simulink model "pure_pursuit"  (R2025b)
settings: Solver=VariableStepAuto  StartTime=0.0  StopTime=40  RelTol=1e-3
libraries: robotmobilelib x2, autolibshared x1
settings Model: Creator=omer  LastModifiedBy=omer

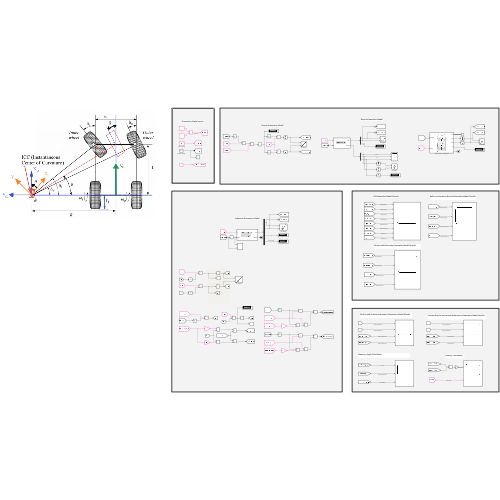
[thumbnail: Simulink's stored preview of the top-level diagram]
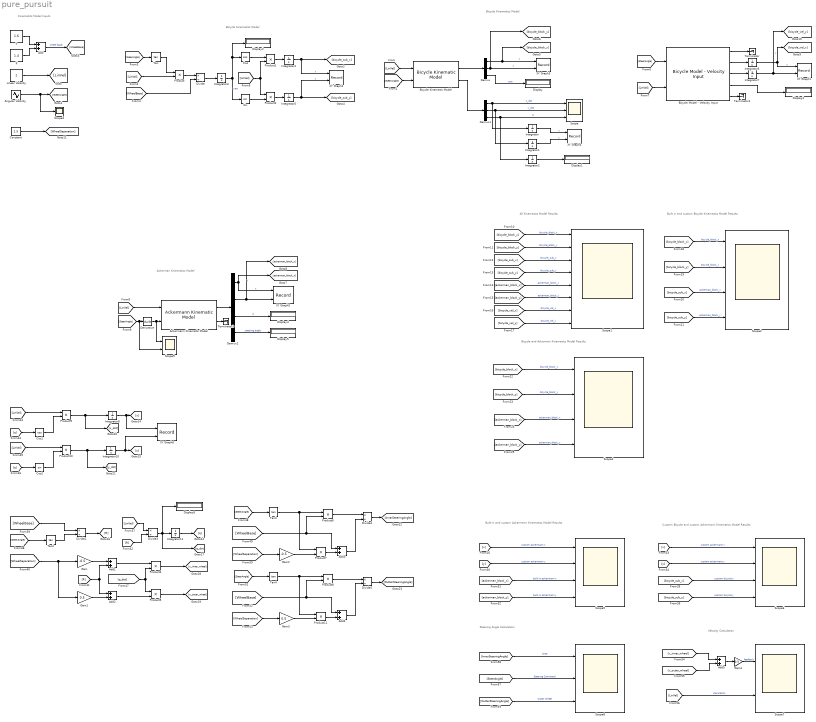
== system pure_pursuit ==
  note: Bicycle Kinematics Model
  note: Bicycle Kinematics Model
  note: Ackerman Kinematics Model
  note: Kinematics Model Inputs
  note: All Kinematics Model Results
  note: Built in and custom Bicycle Kinematics Model Results
  note: Bicycle and Ackerman Kinematics Model Results
  note: Built-in and custom Ackermann Kinematics Model Results
  note: Custom Bicycle and custom Ackermann Kinematics Model Results
  note: Velocity Calculation
  note: Steering Angle Calculation
  Ackermann Kinematic Model : robotmobilelib/Ackermann Kinematic Model  WheelBase=3  VehicleSpeedRange=[-10 10]  MaxSteeringAngle=pi/4  InitialState=[0; 0; 0; 0]  SimulateUsing=Interpreted execution
  Add{,1..5} (6 alike) : Sum
  Angular Velocity : Sin  Amplitude=0.6  Frequency=0.2  SampleTime=0
  Bicycle Kinematic Model : robotmobilelib/Bicycle Kinematic Model  VehicleInputs=Vehicle Speed & Steering Angle  WheelBase=3  VehicleSpeedRange=[-10 10]  MaxSteeringAngle=pi/4  InitialState=[0; 0; 0]  SimulateUsing=Interpreted execution
  Bicycle Model - Velocity Input : autolibshared/Bicycle Model - Velocity Input  trackMode=Single (bicycle)  inputMode=External longitudinal velocity  frontSteerMode=on  rearSteerMode=off  windMode=off  muMode=off  extFMode=off  extMMode=off  aMode=2  NF=2  NR=2  m=2000  a=1.4  b=1.6  h=0.35  X_o=0  xdot_o=0  CalphaMode=off  sigmaMode=on  w=[1.4,1.4]  Cy_f=12e3  Cy_r=11e3  sigma_f=.1  sigma_r=.1  alpha_f_brk=[-.1 .1]  Cy_f_data=[-9e3 9e3]  alpha_r_brk=[-.1 .1]  Cy_r_data=[-9e3 9e3]  Y_o=0  ydot_o=0  Izz=4000  psi_o=0  r_o=0  Af=2  Cd=.3  Cl=.1  Cpm=.1  beta_w=[0 0.01:0.01:0.3]  Cs=[0 0.01:0.01:0.3]  Cym=[0 1e-6:0.01:0.3]  Pabs=101325  Tair=273  g=9.81  mu=1  xdot_tol=.01  Fznom=5000  Fxtire_sat=1e6  Fytire_sat=1e6  longOff=0  latOff=0  vertOff=0
      settings: LibrarySourceBlock=vehdynlibeom/Bicycle Model - Velocity Input
  Constant : Constant  Value=2.5
  Cos : Trigonometry  Operator=cos
  Cos1 : Trigonometry  Operator=cos
  Cos2 : Trigonometry
  Demux : Demux  Outputs=3
  Demux1 : Demux  Outputs=3
  Demux2 : Demux
  Derivative : Derivative
  Display{,1..5,8} (7 alike) : Display
  Divide{,2..5} (5 alike) : Product  Inputs=*/
  Gain : Gain  Gain=-0.5
  Gain1 : Gain  Gain=0.5
  Gain2 : Gain  Gain=-0.5
  Gain3 : Gain  Gain=0.5
  Gain4 : Gain  Gain=0.5
  Integrator{,1..8,10..11} (11 alike) : Integrator
  Linear Velocity : Constant
  Product{,1..2,4..11} (11 alike) : Product
  Scope : Scope  NumInputPorts=3
      settings: ActiveDisplayYMinimum=-1  ActiveDisplayYMaximum=1
  Scope1 : Scope  NumInputPorts=8
      settings: ActiveDisplayYMinimum=-7.1617442519403234  ActiveDisplayYMaximum=20.38246591713515
  Scope{2,4..6} (4 alike) : Scope  NumInputPorts=4
      Scope2 settings: ActiveDisplayYMinimum=0.32572897203293749  ActiveDisplayYMaximum=21.907338374210166  DataLoggingVariableName=ScopeData2
      Scope4 settings: ActiveDisplayYMinimum=32.57770845291958  ActiveDisplayYMaximum=624.63304863060557  DataLoggingVariableName=ScopeData4
      Scope5 settings: ActiveDisplayYMinimum=-4.3902728806219606  ActiveDisplayYMaximum=29.013832851375891  DataLoggingVariableName=ScopeData5
      Scope6 settings: ActiveDisplayYMinimum=-3.4268970997372428  ActiveDisplayYMaximum=28.386536930736913  DataLoggingVariableName=ScopeData6
  Scope3 : Scope
      settings: ActiveDisplayYMinimum=-1.3341695524882851  ActiveDisplayYMaximum=1.7529271348584103  DataLoggingVariableName=ScopeData3
  Scope7 : Scope  NumInputPorts=2
      settings: ActiveDisplayYMinimum=-3.4268970997372428  ActiveDisplayYMaximum=28.386536930736913  DataLoggingVariableName=ScopeData7
  Scope8 : Scope  NumInputPorts=3
      settings: ActiveDisplayYMinimum=-4.3617646340530536  ActiveDisplayYMaximum=11.80186087051403  DataLoggingVariableName=ScopeData8
  Scope9 : Scope  NumInputPorts=2
      settings: ActiveDisplayYMinimum=-1.3341695524882851  ActiveDisplayYMaximum=1.7529271348584103  DataLoggingVariableName=ScopeData9
  Sin : Trigonometry
  Tan{,2..4} (4 alike) : Trigonometry  Operator=tan
  Terminator : Terminator
  Terminator1 : Terminator
  Terminator3 : Terminator
  XY Graph1 : Record  NumPorts=2.0  FileSettingsInternal="{\"entries\":[{\"content\":{\"excelSettings\":{\"content\":{},\"type\":\"Streamout.ExcelSettings\"},\"parquetSettings\":{\"content\":{},\"type\":\"Streamout.ParquetSettings\"}},\"type\":\"Streamout.FileSettingStorage\",\"uuid\":\"\"}],\"packageUris\":[\"http:\\/\\/schema.mathworks.com\\/mf0\\/streamout_blocks\\/R2020a\"],\"version\":\"1.0\"}"  FrameSettings=[0, 0]  Layout=[1 1]  SignalsInternal="{\"entries\":[{\"content\":{\"signals\":[{\"content\":{\"blockPath\":[],\"dimensions\":[1],\"domain\":\"\",\"lineColor\":\"#a2142f\",\"lineWidth\":2,\"plots\":[ 1 ],\"port\":1,\"sid\":[\"\"],\"signalID\":1,\"signalName\":\"x\"},\"type\":\"RecordBlkView.Signal\",\"uuid\":\"\"},{\"content\":{\"blockPath\":[],\"dimensions\":[1],\"domain\":\"\",\"lineColor\":\"#139fff\",\"lineWidth\":2,\"plots\":[ 1 ],\"port\":2,\"sid\":[\"\"],\"signalID\":2,\"signalName\":\"y\"},\"type\":\"RecordBlkView.Signal\",\"uuid\":\"\"}]},\"type\":\"RecordBlkView.InputSignals\",\"uuid\":\"\"}],\"packageUris\":[\"http:\\/\\/schema.mathworks.com\\/mf0\\/streamout_blocks\\/R2020a\"],\"version\":\"1.0\"}"  VisualizationBindings="{\"xyplotplugin\":{\"info\":[{\"series\":[{\"bindingParametersList\":[{\"parameter\":\"X-Axis\",\"signalID\":1,\"signalName\":\"x\"},{\"parameter\":\"Y-Axis\",\"signalID\":2,\"signalName\":\"y\"}],\"seriesID\":0}],\"subplotID\":1}]}}"  CompatibilityTag=XY
  XY Graph2 : Record  NumPorts=2.0  FileSettingsInternal="{\"entries\":[{\"content\":{\"excelSettings\":{\"content\":{},\"type\":\"Streamout.ExcelSettings\"},\"parquetSettings\":{\"content\":{},\"type\":\"Streamout.ParquetSettings\"}},\"type\":\"Streamout.FileSettingStorage\",\"uuid\":\"\"}],\"packageUris\":[\"http:\\/\\/schema.mathworks.com\\/mf0\\/streamout_blocks\\/R2020a\"],\"version\":\"1.0\"}"  FrameSettings=[0, 0]  Layout=[1 1]  SignalsInternal="{\"entries\":[{\"content\":{\"signals\":[{\"content\":{\"blockPath\":[],\"dimensions\":[1],\"domain\":\"\",\"lineColor\":\"#a2142f\",\"plots\":[ 1 ],\"port\":1,\"sid\":[\"\"],\"signalID\":1,\"signalName\":\"x\"},\"type\":\"RecordBlkView.Signal\",\"uuid\":\"\"},{\"content\":{\"blockPath\":[],\"dimensions\":[1],\"domain\":\"\",\"lineColor\":\"#139fff\",\"plots\":[ 1 ],\"port\":2,\"sid\":[\"\"],\"signalID\":2,\"signalName\":\"y\"},\"type\":\"RecordBlkView.Signal\",\"uuid\":\"\"}]},\"type\":\"RecordBlkView.InputSignals\",\"uuid\":\"\"}],\"packageUris\":[\"http:\\/\\/schema.mathworks.com\\/mf0\\/streamout_blocks\\/R2020a\"],\"version\":\"1.0\"}"  VisualizationBindings="{\"xyplotplugin\":{\"info\":[{\"series\":[{\"bindingParametersList\":[{\"parameter\":\"X-Axis\",\"signalID\":1,\"signalName\":\"x\"},{\"parameter\":\"Y-Axis\",\"signalID\":2,\"signalName\":\"y\"}],\"seriesID\":0}],\"subplotID\":1}]}}"  CompatibilityTag=XY
  XY Graph3 : Record  NumPorts=2.0  FileSettingsInternal="{\"entries\":[{\"content\":{\"excelSettings\":{\"content\":{},\"type\":\"Streamout.ExcelSettings\"},\"parquetSettings\":{\"content\":{},\"type\":\"Streamout.ParquetSettings\"}},\"type\":\"Streamout.FileSettingStorage\",\"uuid\":\"\"}],\"packageUris\":[\"http:\\/\\/schema.mathworks.com\\/mf0\\/streamout_blocks\\/R2020a\"],\"version\":\"1.0\"}"  FrameSettings=[0, 0]  Layout=[1 1]  SignalsInternal="{\"entries\":[{\"content\":{\"signals\":[{\"content\":{\"blockPath\":[],\"dimensions\":[1],\"domain\":\"\",\"lineColor\":\"#a2142f\",\"plots\":[ 1 ],\"port\":1,\"sid\":[\"\"],\"signalID\":1,\"signalName\":\"x\"},\"type\":\"RecordBlkView.Signal\",\"uuid\":\"\"},{\"content\":{\"blockPath\":[],\"dimensions\":[1],\"domain\":\"\",\"lineColor\":\"#139fff\",\"plots\":[ 1 ],\"port\":2,\"sid\":[\"\"],\"signalID\":2,\"signalName\":\"y\"},\"type\":\"RecordBlkView.Signal\",\"uuid\":\"\"}]},\"type\":\"RecordBlkView.InputSignals\",\"uuid\":\"\"}],\"packageUris\":[\"http:\\/\\/schema.mathworks.com\\/mf0\\/streamout_blocks\\/R2020a\"],\"version\":\"1.0\"}"  VisualizationBindings="{\"xyplotplugin\":{\"info\":[{\"series\":[{\"bindingParametersList\":[{\"parameter\":\"X-Axis\",\"signalID\":1,\"signalName\":\"x\"},{\"parameter\":\"Y-Axis\",\"signalID\":2,\"signalName\":\"y\"}],\"seriesID\":0}],\"subplotID\":1}]}}"  CompatibilityTag=XY
  XY Graph4 : Record  NumPorts=2.0  FileSettingsInternal="{\"entries\":[{\"content\":{\"excelSettings\":{\"content\":{},\"type\":\"Streamout.ExcelSettings\"},\"parquetSettings\":{\"content\":{},\"type\":\"Streamout.ParquetSettings\"}},\"type\":\"Streamout.FileSettingStorage\",\"uuid\":\"\"}],\"packageUris\":[\"http:\\/\\/schema.mathworks.com\\/mf0\\/streamout_blocks\\/R2020a\"],\"version\":\"1.0\"}"  FrameSettings=[0, 0]  Layout=[1 1]  SignalsInternal="{\"entries\":[{\"content\":{\"signals\":[{\"content\":{\"blockPath\":[],\"dimensions\":[1],\"domain\":\"\",\"lineColor\":\"#a2142f\",\"lineWidth\":2,\"plots\":[ 1 ],\"port\":1,\"sid\":[\"\"],\"signalID\":1,\"signalName\":\"x\"},\"type\":\"RecordBlkView.Signal\",\"uuid\":\"\"},{\"content\":{\"blockPath\":[],\"dimensions\":[1],\"domain\":\"\",\"lineColor\":\"#139fff\",\"lineWidth\":2,\"plots\":[ 1 ],\"port\":2,\"sid\":[\"\"],\"signalID\":2,\"signalName\":\"y\"},\"type\":\"RecordBlkView.Signal\",\"uuid\":\"\"}]},\"type\":\"RecordBlkView.InputSignals\",\"uuid\":\"\"}],\"packageUris\":[\"http:\\/\\/schema.mathworks.com\\/mf0\\/streamout_blocks\\/R2020a\"],\"version\":\"1.0\"}"  VisualizationBindings="{\"xyplotplugin\":{\"info\":[{\"series\":[{\"bindingParametersList\":[{\"parameter\":\"X-Axis\",\"signalID\":1,\"signalName\":\"x\"},{\"parameter\":\"Y-Axis\",\"signalID\":2,\"signalName\":\"y\"}],\"seriesID\":0}],\"subplotID\":1}]}}"  CompatibilityTag=XY
  XY Graph5 : Record  NumPorts=2.0  FileSettingsInternal="{\"entries\":[{\"content\":{\"excelSettings\":{\"content\":{},\"type\":\"Streamout.ExcelSettings\"},\"parquetSettings\":{\"content\":{},\"type\":\"Streamout.ParquetSettings\"}},\"type\":\"Streamout.FileSettingStorage\",\"uuid\":\"\"}],\"packageUris\":[\"http:\\/\\/schema.mathworks.com\\/mf0\\/streamout_blocks\\/R2020a\"],\"version\":\"1.0\"}"  FrameSettings=[0, 0]  Layout=[1 1]  SignalsInternal="{\"entries\":[{\"content\":{\"signals\":[{\"content\":{\"blockPath\":[],\"dimensions\":[1],\"domain\":\"\",\"lineColor\":\"#a2142f\",\"lineWidth\":2,\"plots\":[ 1 ],\"port\":1,\"sid\":[\"\"],\"signalID\":1,\"signalName\":\"x\"},\"type\":\"RecordBlkView.Signal\",\"uuid\":\"\"},{\"content\":{\"blockPath\":[],\"dimensions\":[1],\"domain\":\"\",\"lineColor\":\"#139fff\",\"plots\":[ 1 ],\"port\":2,\"sid\":[\"\"],\"signalID\":2,\"signalName\":\"y\"},\"type\":\"RecordBlkView.Signal\",\"uuid\":\"\"}]},\"type\":\"RecordBlkView.InputSignals\",\"uuid\":\"\"}],\"packageUris\":[\"http:\\/\\/schema.mathworks.com\\/mf0\\/streamout_blocks\\/R2020a\"],\"version\":\"1.0\"}"  VisualizationBindings="{\"xyplotplugin\":{\"info\":[{\"series\":[{\"bindingParametersList\":[{\"parameter\":\"X-Axis\",\"signalID\":1,\"signalName\":\"x\"},{\"parameter\":\"Y-Axis\",\"signalID\":2,\"signalName\":\"y\"}],\"seriesID\":0}],\"subplotID\":1}]}}"  CompatibilityTag=XY
  XY Graph6 : Record  NumPorts=2.0  FileSettingsInternal="{\"entries\":[{\"content\":{\"excelSettings\":{\"content\":{},\"type\":\"Streamout.ExcelSettings\"},\"parquetSettings\":{\"content\":{},\"type\":\"Streamout.ParquetSettings\"}},\"type\":\"Streamout.FileSettingStorage\",\"uuid\":\"\"}],\"packageUris\":[\"http:\\/\\/schema.mathworks.com\\/mf0\\/streamout_blocks\\/R2020a\"],\"version\":\"1.0\"}"  FrameSettings=[0, 0]  Layout=[1 1]  SignalsInternal="{\"entries\":[{\"content\":{\"signals\":[{\"content\":{\"blockPath\":[],\"dimensions\":[1],\"domain\":\"\",\"lineColor\":\"#a2142f\",\"lineWidth\":2,\"plots\":[ 1 ],\"port\":1,\"sid\":[\"\"],\"signalID\":1,\"signalName\":\"Integrator8\"},\"type\":\"RecordBlkView.Signal\",\"uuid\":\"\"},{\"content\":{\"blockPath\":[],\"dimensions\":[1],\"domain\":\"\",\"lineColor\":\"#139fff\",\"plots\":[ 1 ],\"port\":2,\"sid\":[\"\"],\"signalID\":2,\"signalName\":\"Integrator10\"},\"type\":\"RecordBlkView.Signal\",\"uuid\":\"\"}]},\"type\":\"RecordBlkView.InputSignals\",\"uuid\":\"\"}],\"packageUris\":[\"http:\\/\\/schema.mathworks.com\\/mf0\\/streamout_blocks\\/R2020a\"],\"version\":\"1.0\"}"  VisualizationBindings="{\"xyplotplugin\":{\"info\":[{\"series\":[{\"bindingParametersList\":[{\"parameter\":\"X-Axis\",\"signalID\":1,\"signalName\":\"Integrator8\"},{\"parameter\":\"Y-Axis\",\"signalID\":2,\"signalName\":\"Integrator10\"}],\"seriesID\":0}],\"subplotID\":1}]}}"  CompatibilityTag=XY
  lf : Constant  Value=1.4
  lr : Constant  Value=1.6
  wires:
  Bicycle Kinematic Model/2 -> Demux1/1
  Bicycle Kinematic Model/1 -> Demux/1
  Demux/1 -> [bicycle_block_x], XY Graph3/1  "x"
  Demux/2 -> [bicycle_block_y], XY Graph3/2  "y"
  Demux/3 -> Display/1  "yaw"
  Demux1/1 -> Integrator/1, Scope/1  "x_dot"
  Demux1/2 -> Integrator1/1, Scope/2  "y_dot"
  Demux1/3 -> Integrator2/1, Scope/3  "w"
  Integrator2/1 -> Display1/1
  Integrator/1 -> XY Graph4/1  "x"
  Integrator1/1 -> XY Graph4/2  "y"
  Linear Velocity/1 -> [LinVel]
  [LinVel] -> Bicycle Kinematic Model/1
  [SteerAngle] -> Bicycle Kinematic Model/2
  lr/1 -> Add/1
  lf/1 -> Add/2
  Add/1 -> [WheelBase]  "wheel base"
  [SteerAngle] -> Tan/1
  Tan/1 -> Product/1
  [LinVel] -> Product/2
  Product/1 -> Divide/1
  [WheelBase] -> Divide/2
  Divide/1 -> Integrator3/1
  Integrator3/1 -> Display2/1, Cos/1, Sin/1  "yaw"
  Cos/1 -> Product1/1
  Sin/1 -> Product2/2
  [LinVel] -> Product2/1, Product1/2
  Product1/1 -> Integrator4/1
  Product2/1 -> Integrator5/1
  Integrator4/1 -> [bicycle_sub_x], XY Graph2/1  "x"
  Integrator5/1 -> XY Graph2/2, [bicycle_sub_y]  "y"
  [SteerAngle] -> Bicycle Model - Velocity Input/1
  [LinVel] -> Bicycle Model - Velocity Input/2
  Bicycle Model - Velocity Input/1 -> Terminator/1
  Bicycle Model - Velocity Input/2 -> Integrator6/1
  Bicycle Model - Velocity Input/3 -> Integrator7/1
  Bicycle Model - Velocity Input/4 -> Display3/1
  Integrator6/1 -> [bicycle_vel_x], XY Graph1/1  "x"
  Integrator7/1 -> [bicycle_vel_y], XY Graph1/2  "y"
  Bicycle Model - Velocity Input/5 -> Terminator1/1
  [LinVel] -> Ackermann Kinematic Model/1
  [SteerAngle] -> Scope9/2, Derivative/1
  Derivative/1 -> Scope9/1, Ackermann Kinematic Model/2
  Ackermann Kinematic Model/1 -> Demux2/1
  Demux2/1 -> XY Graph5/1, [ackerman_block_x]  "x"
  Demux2/2 -> [ackerman_block_y], XY Graph5/2  "y"
  Demux2/3 -> Display4/1  "q"
  Ackermann Kinematic Model/2 -> Terminator3/1
  Demux2/4 -> Display5/1  "steering angle"
  Angular Velocity/1 -> Scope3/1, [SteerAngle]
  [bicycle_block_x] -> Scope1/1  "bicycle_block_x"
  [bicycle_block_y] -> Scope1/2  "bicycle_block_y"
  [bicycle_sub_x] -> Scope1/3  "bicycle_sub_x"
  [bicycle_sub_y] -> Scope1/4  "bicycle_sub_y"
  [ackerman_block_x] -> Scope1/5  "ackerman_block_x"
  [ackerman_block_y] -> Scope1/6  "ackerman_block_y"
  [bicycle_vel_x] -> Scope1/7  "bicycle_vel_x"
  [bicycle_vel_y] -> Scope1/8  "bicycle_vel_y"
  [bicycle_block_x] -> Scope2/1  "bicycle_block_x"
  [bicycle_block_y] -> Scope2/2  "bicycle_block_y"
  [bicycle_sub_x] -> Scope2/3  "ackerman_block_x"
  [bicycle_sub_y] -> Scope2/4  "ackerman_block_y"
  [ackerman_block_y] -> Scope4/4  "ackerman_block_y"
  [bicycle_block_x] -> Scope4/1  "bicycle_block_x"
  [bicycle_block_y] -> Scope4/2  "bicycle_block_y"
  [ackerman_block_x] -> Scope4/3  "ackerman_block_x"
  [LinVel] -> Product9/1
  [q] -> Cos1/1
  Cos1/1 -> Product9/2
  Cos2/1 -> Product10/2
  [LinVel] -> Product10/1
  [q] -> Cos2/1
  Product9/1 -> [x_dot], Integrator8/1
  Product10/1 -> [y_dot], Integrator10/1
  Integrator8/1 -> XY Graph6/1, [x]
  Integrator10/1 -> XY Graph6/2, [y]
  [x] -> Scope5/1  "custom ackermann x"
  [y] -> Scope5/2  "custom ackermann y"
  [ackerman_block_x] -> Scope5/3  "built-in ackermann x"
  [ackerman_block_y] -> Scope5/4  "built-in ackermann y"
  [y] -> Scope6/2  "custom ackermann y"
  [x] -> Scope6/1  "custom ackermann x"
  [bicycle_sub_y] -> Scope6/4  "custom bicycle y"
  [bicycle_sub_x] -> Scope6/3  "custom bicycle x"
  Constant/1 -> [WheelSeparation]
  [SteerAngle] -> Tan2/1
  Tan2/1 -> Divide2/2
  Divide2/1 -> [R]
  [WheelBase] -> Divide2/1
  [WheelSeparation] -> Gain1/1, Gain/1
  Gain/1 -> Add1/1
  [R] -> Add2/1, Add1/2
  Gain1/1 -> Add2/2
  [LinVel] -> Divide3/1
  [R] -> Divide3/2
  Divide3/1 -> [q_dot], Integrator11/1, Display8/1
  Add1/1 -> Product4/1
  [q_dot] -> Product5/1, Product4/2
  Add2/1 -> Product5/2
  Product4/1 -> [v_inner_wheel]
  Product5/1 -> [v_outer_wheel]
  [SteerAngle] -> Tan3/1
  Tan3/1 -> Product7/1, Product6/1
  [WheelBase] -> Add3/1, Product6/2
  Product6/1 -> Divide4/1
  [WheelSeparation] -> Gain2/1
  Gain2/1 -> Product7/2
  Product7/1 -> Add3/2
  Add3/1 -> Divide4/2
  Divide4/1 -> [InnerSteeringAngle]
  Product11/1 -> Add4/2
  [SteerAngle] -> Tan4/1
  Product8/1 -> Divide5/1
  [WheelBase] -> Add4/1, Product8/2
  Divide5/1 -> [OutterSteeringAngle]
  Gain3/1 -> Product11/2
  Add4/1 -> Divide5/2
  [WheelSeparation] -> Gain3/1
  Tan4/1 -> Product11/1, Product8/1
  [v_inner_wheel] -> Add5/1
  [v_outer_wheel] -> Add5/2
  Add5/1 -> Gain4/1
  Gain4/1 -> Scope7/1  "feedback"
  [LinVel] -> Scope7/2  "calculation"
  [InnerSteeringAngle] -> Scope8/1  "Inner"
  [SteerAngle] -> Scope8/2  "Steerıng Command"
  [OutterSteeringAngle] -> Scope8/3  "Outer Wheel"
  Integrator11/1 -> [q]
